simulink model "pi_IL_H2DF_2024a"  (R2024a)
settings: Solver=FixedStepAuto  StartTime=0.0  StopTime=inf  FixedStep=0.001  RelTol=1e-3  EnableMultiTasking=on
values from neighbouring files (symbols this model uses):
  IL = struct()    [init_simulink_IL_H2DF.m]
undefined symbols (not defined in the file or in its folder): C2C_NMPC
libraries: deeplib x1, raspberrypiNetworklib x1
(part 1 of 2)
settings Model: VariantConfigurationObject=C2C  SimulationMode=external  ExtModeTrigDuration=2  Creator=maxim  LastModifiedBy=winkler_a
settings SolverCC: PositivePriorityOrder=on
settings DataIOCC: LimitDataPoints=on  MaxDataPoints=10000  SaveOutput=off
settings OptimizationCC: EnhancedBackFolding=on  PassReuseOutputArgsAs=Individual arguments  ZeroExternalMemoryAtStartup=off  ZeroInternalMemoryAtStartup=off  MaxStackSize=64  OptimizeBlockOrder=speed  DifferentSizesBufferReuse=on  OptimizationCustomize=off  EfficientTunableParamExpr=on
settings DebuggingCC: ParameterTunabilityLossMsg=error
settings HardwareCC: ProdBitPerPointer=32  ProdBitPerSizeT=32  ProdBitPerPtrDiffT=32  ProdLargestAtomicInteger=Long  ProdLargestAtomicFloat=Double  ProdWordSize=32  ProdLongLongMode=on  ProdHWDeviceType=ARM Compatible->ARM Cortex
settings RTWCC: Description=Embedded Coder  SystemTargetFile=ert.tlc  HardwareBoard=Raspberry Pi  TemplateMakefile=ert_default_tmf  RTWUseSimCustomCode=on  Toolchain=GNU GCC Embedded Linux  BuildConfiguration=Faster Runs  GPUComputeCapability=3.5
settings CodeAppCC: ForceParamTrailComments=on  IgnoreCustomStorageClasses=off  OperatorAnnotations=on  SimulinkDataObjDesc=on  SFDataObjDesc=on  InsertBlockDesc=on
settings ERTTargetCC: SupportContinuousTime=on  SupportNonInlinedSFcns=on  SupportVariableSizeSignals=on  ExtMode=on  ExtModeStaticAlloc=on  ExtModeMaxTrigDuration=1000  ExtModeMexArgs='192.168.140.200' 0 17725

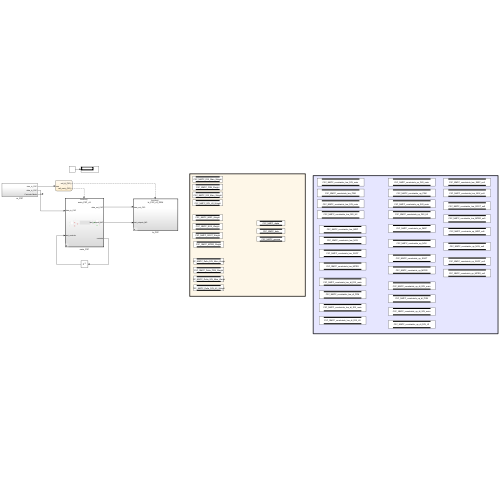
[thumbnail: Simulink's stored preview of the top-level diagram]
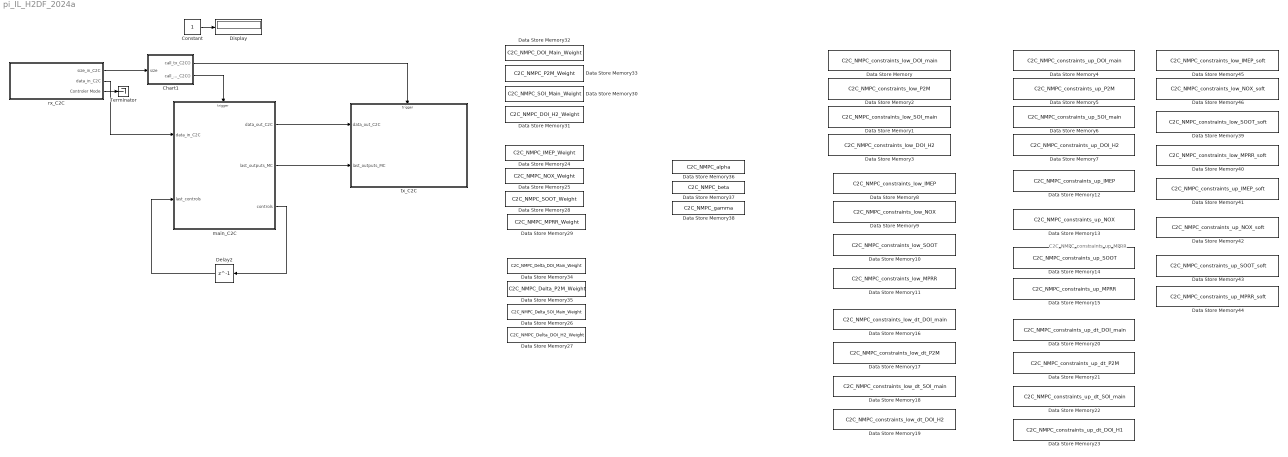
== system pi_IL_H2DF_2024a ==
  note: C2C_NMPC_constraints_up_MPRR
  Chart1 : Stateflow chart  TreatAsAtomicUnit=on
  Constant : Constant
  Data Store Memory : DataStoreMemory  DataStoreName=C2C_NMPC_constraints_low_DOI_main  WriteAfterWriteMsg=warning  ShowAdditionalParam=off
  Data Store Memory1 : DataStoreMemory  DataStoreName=C2C_NMPC_constraints_low_SOI_main  WriteAfterWriteMsg=warning  ShowAdditionalParam=off
  Data Store Memory10 : DataStoreMemory  DataStoreName=C2C_NMPC_constraints_low_SOOT  WriteAfterWriteMsg=warning  ShowAdditionalParam=off
  Data Store Memory11 : DataStoreMemory  DataStoreName=C2C_NMPC_constraints_low_MPRR  WriteAfterWriteMsg=warning  ShowAdditionalParam=off
  Data Store Memory12 : DataStoreMemory  DataStoreName=C2C_NMPC_constraints_up_IMEP  WriteAfterWriteMsg=warning  ShowAdditionalParam=off
  Data Store Memory13 : DataStoreMemory  DataStoreName=C2C_NMPC_constraints_up_NOX  WriteAfterWriteMsg=warning  ShowAdditionalParam=off
  Data Store Memory14 : DataStoreMemory  DataStoreName=C2C_NMPC_constraints_up_SOOT  WriteAfterWriteMsg=warning  ShowAdditionalParam=off
  Data Store Memory15 : DataStoreMemory  DataStoreName=C2C_NMPC_constraints_up_MPRR  WriteAfterWriteMsg=warning  ShowAdditionalParam=off
  Data Store Memory16 : DataStoreMemory  DataStoreName=C2C_NMPC_constraints_low_dt_DOI_main  WriteAfterWriteMsg=warning  ShowAdditionalParam=off
  Data Store Memory17 : DataStoreMemory  DataStoreName=C2C_NMPC_constraints_low_dt_P2M  WriteAfterWriteMsg=warning  ShowAdditionalParam=off
  Data Store Memory18 : DataStoreMemory  DataStoreName=C2C_NMPC_constraints_low_dt_SOI_main  WriteAfterWriteMsg=warning  ShowAdditionalParam=off
  Data Store Memory19 : DataStoreMemory  DataStoreName=C2C_NMPC_constraints_low_dt_DOI_H2  WriteAfterWriteMsg=warning  ShowAdditionalParam=off
  Data Store Memory2 : DataStoreMemory  DataStoreName=C2C_NMPC_constraints_low_P2M  WriteAfterWriteMsg=warning  ShowAdditionalParam=off
  Data Store Memory20 : DataStoreMemory  DataStoreName=C2C_NMPC_constraints_up_dt_DOI_main  WriteAfterWriteMsg=warning  ShowAdditionalParam=off
  Data Store Memory21 : DataStoreMemory  DataStoreName=C2C_NMPC_constraints_up_dt_P2M  WriteAfterWriteMsg=warning  ShowAdditionalParam=off
  Data Store Memory22 : DataStoreMemory  DataStoreName=C2C_NMPC_constraints_up_dt_SOI_main  WriteAfterWriteMsg=warning  ShowAdditionalParam=off
  Data Store Memory23 : DataStoreMemory  DataStoreName=C2C_NMPC_constraints_up_dt_DOI_H1  WriteAfterWriteMsg=warning  ShowAdditionalParam=off
  Data Store Memory24 : DataStoreMemory  DataStoreName=C2C_NMPC_IMEP_Weight  WriteAfterWriteMsg=warning  ShowAdditionalParam=off
  Data Store Memory25 : DataStoreMemory  DataStoreName=C2C_NMPC_NOX_Weight  WriteAfterWriteMsg=warning  ShowAdditionalParam=off
  Data Store Memory26 : DataStoreMemory  DataStoreName=C2C_NMPC_Delta_SOI_Main_Weight  WriteAfterWriteMsg=warning  ShowAdditionalParam=off
  Data Store Memory27 : DataStoreMemory  DataStoreName=C2C_NMPC_Delta_DOI_H2_Weight  WriteAfterWriteMsg=warning  ShowAdditionalParam=off
  Data Store Memory28 : DataStoreMemory  DataStoreName=C2C_NMPC_SOOT_Weight  WriteAfterWriteMsg=warning  ShowAdditionalParam=off
  Data Store Memory29 : DataStoreMemory  DataStoreName=C2C_NMPC_MPRR_Weight  WriteAfterWriteMsg=warning  ShowAdditionalParam=off
  Data Store Memory3 : DataStoreMemory  DataStoreName=C2C_NMPC_constraints_low_DOI_H2  WriteAfterWriteMsg=warning  ShowAdditionalParam=off
  Data Store Memory30 : DataStoreMemory  DataStoreName=C2C_NMPC_SOI_Main_Weight  WriteAfterWriteMsg=warning  ShowAdditionalParam=off
  Data Store Memory31 : DataStoreMemory  DataStoreName=C2C_NMPC_DOI_H2_Weight  WriteAfterWriteMsg=warning  ShowAdditionalParam=off
  Data Store Memory32 : DataStoreMemory  DataStoreName=C2C_NMPC_DOI_Main_Weight  WriteAfterWriteMsg=warning  ShowAdditionalParam=off
  Data Store Memory33 : DataStoreMemory  DataStoreName=C2C_NMPC_P2M_Weight  WriteAfterWriteMsg=warning  ShowAdditionalParam=off
  Data Store Memory34 : DataStoreMemory  DataStoreName=C2C_NMPC_Delta_DOI_Main_Weight  WriteAfterWriteMsg=warning  ShowAdditionalParam=off
  Data Store Memory35 : DataStoreMemory  DataStoreName=C2C_NMPC_Delta_P2M_Weight  WriteAfterWriteMsg=warning  ShowAdditionalParam=off
  Data Store Memory36 : DataStoreMemory  DataStoreName=C2C_NMPC_alpha  WriteAfterWriteMsg=warning  ShowAdditionalParam=off
  Data Store Memory37 : DataStoreMemory  DataStoreName=C2C_NMPC_beta  WriteAfterWriteMsg=warning  ShowAdditionalParam=off
  Data Store Memory38 : DataStoreMemory  DataStoreName=C2C_NMPC_gamma  WriteAfterWriteMsg=warning  ShowAdditionalParam=off
  Data Store Memory39 : DataStoreMemory  DataStoreName=C2C_NMPC_constraints_low_SOOT_soft  WriteAfterWriteMsg=warning  ShowAdditionalParam=off
  Data Store Memory4 : DataStoreMemory  DataStoreName=C2C_NMPC_constraints_up_DOI_main  WriteAfterWriteMsg=warning  ShowAdditionalParam=off
  Data Store Memory40 : DataStoreMemory  DataStoreName=C2C_NMPC_constraints_low_MPRR_soft  WriteAfterWriteMsg=warning  ShowAdditionalParam=off
  Data Store Memory41 : DataStoreMemory  DataStoreName=C2C_NMPC_constraints_up_IMEP_soft  WriteAfterWriteMsg=warning  ShowAdditionalParam=off
  Data Store Memory42 : DataStoreMemory  DataStoreName=C2C_NMPC_constraints_up_NOX_soft  WriteAfterWriteMsg=warning  ShowAdditionalParam=off
  Data Store Memory43 : DataStoreMemory  DataStoreName=C2C_NMPC_constraints_up_SOOT_soft  WriteAfterWriteMsg=warning  ShowAdditionalParam=off
  Data Store Memory44 : DataStoreMemory  DataStoreName=C2C_NMPC_constraints_up_MPRR_soft  WriteAfterWriteMsg=warning  ShowAdditionalParam=off
  Data Store Memory45 : DataStoreMemory  DataStoreName=C2C_NMPC_constraints_low_IMEP_soft  WriteAfterWriteMsg=warning  ShowAdditionalParam=off
  Data Store Memory46 : DataStoreMemory  DataStoreName=C2C_NMPC_constraints_low_NOX_soft  WriteAfterWriteMsg=warning  ShowAdditionalParam=off
  Data Store Memory5 : DataStoreMemory  DataStoreName=C2C_NMPC_constraints_up_P2M  WriteAfterWriteMsg=warning  ShowAdditionalParam=off
  Data Store Memory6 : DataStoreMemory  DataStoreName=C2C_NMPC_constraints_up_SOI_main  WriteAfterWriteMsg=warning  ShowAdditionalParam=off
  Data Store Memory7 : DataStoreMemory  DataStoreName=C2C_NMPC_constraints_up_DOI_H2  WriteAfterWriteMsg=warning  ShowAdditionalParam=off
  Data Store Memory8 : DataStoreMemory  DataStoreName=C2C_NMPC_constraints_low_IMEP  WriteAfterWriteMsg=warning  ShowAdditionalParam=off
  Data Store Memory9 : DataStoreMemory  DataStoreName=C2C_NMPC_constraints_low_NOX  WriteAfterWriteMsg=warning  ShowAdditionalParam=off
  Delay2 : Delay  DelayLength=1  InitialCondition=C2C_NMPC.x0([(C2C_NMPC.Dims.n_LSTM_states + 1):(C2C_NMPC.Dims.n_LSTM_states + C2C_NMPC.Dims.n_controls)])
  Display : Display
  Terminator : Terminator
  main_C2C : Subsystem  Variant=on  VariantControlMode=label  VariantControl=main_C2C_n3  LabelModeActiveChoice=main_C2C_n3
  rx_C2C : Subsystem
  tx_C2C : Subsystem  Variant=on  VariantControlMode=label  VariantControl=Choice  LabelModeActiveChoice=tx_C2C_n3_GRU
  wires:
  rx_C2C/1(size_in_C2C) -> Chart1/1(size)
  Chart1/1(call_tx_C2C()) -> tx_C2C/Trigger
  rx_C2C/2(data_in_C2C) -> main_C2C/1(data_in_C2C)
  Delay2/1 -> main_C2C/2(last_controls)
  Chart1/2(call_main_C2C()) -> main_C2C/Trigger
  main_C2C/1(data_out_C2C) -> tx_C2C/1(data_out_C2C)
  main_C2C/3(controls) -> Delay2/1
  main_C2C/2(last_outputs_MC) -> tx_C2C/2(last_outputs_MC)
  Constant/1 -> Display/1
  rx_C2C/3(Controler Mode) -> Terminator/1

== system pi_IL_H2DF_2024a/main_C2C ==
  data_in_C2C : Inport
  last_controls : Inport  Port=2
  function : TriggerPort  TriggerType=function-call  VariantControl=(inherit)
  main_C2C_n3 : Subsystem  VariantControl=main_C2C_n3
  data_out_C2C : Outport
  last_outputs_MC : Outport  Port=2
  controls : Outport  Port=3

== system pi_IL_H2DF_2024a/rx_C2C ==
  Data Type Conversion : DataTypeConversion  OutDataTypeStr=double  SaturateOnIntegerOverflow=off  RndMeth=Floor
  Receive : Subsystem
  UDP Receive1 : raspberrypiNetworklib/UDP Receive  localURL='0.0.0.0'  localPort=42785  remoteURL='0.0.0.0'  remotePort=-1  recvBufferSize=8192  signalDatatype=uint32  dims=56  isVarSize=off  showBlockingTime=off  blockingTime=0  sampletime=0.001  blockPlatform=Raspberry Pi
  size_in_C2C : Outport
  data_in_C2C : Outport  Port=2
  Controler Mode : Outport  Port=3
  wires:
  UDP Receive1/2 -> size_in_C2C/1
  UDP Receive1/1 -> Data Type Conversion/1
  Receive/1(udp_outputs) -> data_in_C2C/1
  Data Type Conversion/1 -> Receive/1(udp_data_in)
  Receive/2(controller_mode) -> Controler Mode/1

== system pi_IL_H2DF_2024a/tx_C2C ==
  data_out_C2C : Inport
  last_outputs_MC : Inport  Port=2
  function : TriggerPort  TriggerType=function-call  VariantControl=(inherit)
  tx_C2C_n3_GRU : Subsystem  VariantControl=tx_C2C_n3_GRU

== system pi_IL_H2DF_2024a/main_C2C/main_C2C_n3 ==
  data_in_C2C : Inport
  last_controls : Inport  Port=2
  function : TriggerPort  TriggerType=function-call  VariantControl=(inherit)
  Constant : Constant  Value=zeros(16,1)
  IC : InitialCondition  Value=C2C_NMPC.x0([(C2C_NMPC.Dims.n_LSTM_states + 1):(C2C_NMPC.Dims.n_LSTM_states + C2C_NMPC.Dims.n_controls)])
  IL_Controller : Subsystem  VariantControl=C2C_NMPC_n3
  Selector : Selector  InputPortWidth=C2C_NMPC.Dims.n_cost*3  IndexOptions=Index vector (dialog)  Indices=1:C2C_NMPC.Dims.n_cost  OutputSizes=1
  post_processing : Subsystem
  pre_processing1 : Subsystem
  data_out_C2C : Outport
  last_outputs_MC : Outport  Port=2
  controls : Outport  Port=3
  wires:
  post_processing/1(data_C2C_out) -> data_out_C2C/1
  pre_processing1/1(reference_C2C) -> IL_Controller/1(reference_C2C), Selector/1
  pre_processing1/2(counter_C2C) -> [counter_C2C]
  [counter_C2C] -> post_processing/5(counter)
  last_controls/1 -> [last_controls]
  IL_Controller/1(status_C2C) -> post_processing/3(controller_status)
  [last_outputs_MC] -> post_processing/4(last_outputs_MC)
  [last_outputs_MC] -> last_outputs_MC/1
  pre_processing1/3(last_outputs_MC) -> IL_Controller/2(last_outputs), [last_outputs_MC]
  data_in_C2C/1 -> pre_processing1/1(data_in_C2C)
  Selector/1 -> post_processing/1(reference)
  IL_Controller/2(controls) -> IC/1
  IC/1 -> post_processing/2(controls), controls/1
  Constant/1 -> post_processing/6(LSTM_States)

== system pi_IL_H2DF_2024a/rx_C2C/Receive ==
  note: block for horizon of 3 from engine
  udp_data_in : Inport
  conversion_n3 : Subsystem
  udp_outputs : Outport
  controller_mode : Outport  Port=2
  wires:
  udp_data_in/1 -> conversion_n3/1(udp_data_in)
  conversion_n3/1(udp_outputs) -> udp_outputs/1
  conversion_n3/2(controller_mode) -> controller_mode/1

== system pi_IL_H2DF_2024a/tx_C2C/tx_C2C_n3_GRU ==
  note: [1:4,13,99:134,14,15,16,17,71:74]
  data_out_C2C : Inport
  last_outputs_MC : Inport  Port=2
  function : TriggerPort  TriggerType=function-call  VariantControl=(inherit)
  Data Type Conversion : DataTypeConversion  OutDataTypeStr=uint32  SaturateOnIntegerOverflow=off  RndMeth=Floor
  Selector : Selector  IndexOptions=Index vector (dialog)  Indices=[1:4,13,115:142,14,15,16,17,95:98]  OutputSizes=1
  Subsystem : Subsystem
  UDP Send1 : S-Function  AncestorBlock=raspberrypiNetworklib/UDP Send  InitFcn=|  FunctionName=sdspToNetwork  Parameters=localURL, localPortSource, localPort, remoteURL, remotePort, 8192, separateLengthPort, []  SFunctionDeploymentMode=off  EnableBusSupport=off  mask(UDP Send){remoteURL='192.168.140.159', remotePort=42784, localURL='0.0.0.0', localPortSource=Specify via dialog, localPort=42784, sampletime=-1, blockPlatform=Raspberry Pi, separateLengthPort=0}
      | realtime.internal.validateLinuxBlock(get_param(gcbh, 'blockPlatform'), gcbh);
      | realtime.internal.registerLinuxBlock(gcb);
      mask prompts: remoteURL "Remote IP address ('255.255.255.255' for broadcast):"; remotePort "Remote IP port:"; localURL "Local IP address:"; localPortSource "Local IP port source:"; localPort "Local IP port:"; blockPlatform "Block Platform"; separateLengthPort "Use a separate length port"
      mask help: Sends UDP packets to another UDP host on an Internet network. Set Remote IP address parameter to the IP address of the receiving UDP host. Set the Remote IP port parameter to the port number used by the receiving UDP host.
      settings: LibrarySourceBlock=raspberrypiNetworklib/UDP Send
      mask Help: eval('realtime.helpView(get_param(gcb, ''blockPlatform''), [realtime.internal.getHelpLinkPrefix(gcb) ''libudpsend''])');
      mask TypeOptions localPortSource: Automatically determine | Specify via dialog
      mask Callback localPortSource:
      | mask_vis = get_param(gcbh, 'MaskVisibilities');
      | if strcmp(get_param(gcbh,'localPortSource'),'Specify via dialog')
      |     mask_vis{5} = 'on';
      | else
      |     mask_vis{5} = 'off';
      | end
      | set_param(gcbh, 'MaskVisibilities', mask_vis);
      | clear('mask_vis');
      mask Display:
      | %fprintf('UDP Send');
      | color('blue');
      | [data, map]=imread('ethernet2_bw.gif');pic=ind2rgb(data,map);image(pic,[0.32 0.25 0.40 0.45]);
      | platform = realtime.internal.getBlockDisplayText(gcb);
      | text(0.99, 0.9, platform, 'horizontalalignment', 'right');
  wires:
  data_out_C2C/1 -> Selector/1
  Data Type Conversion/1 -> UDP Send1/1
  Subsystem/1(Out1) -> Data Type Conversion/1
  Selector/1 -> Subsystem/1(In1)

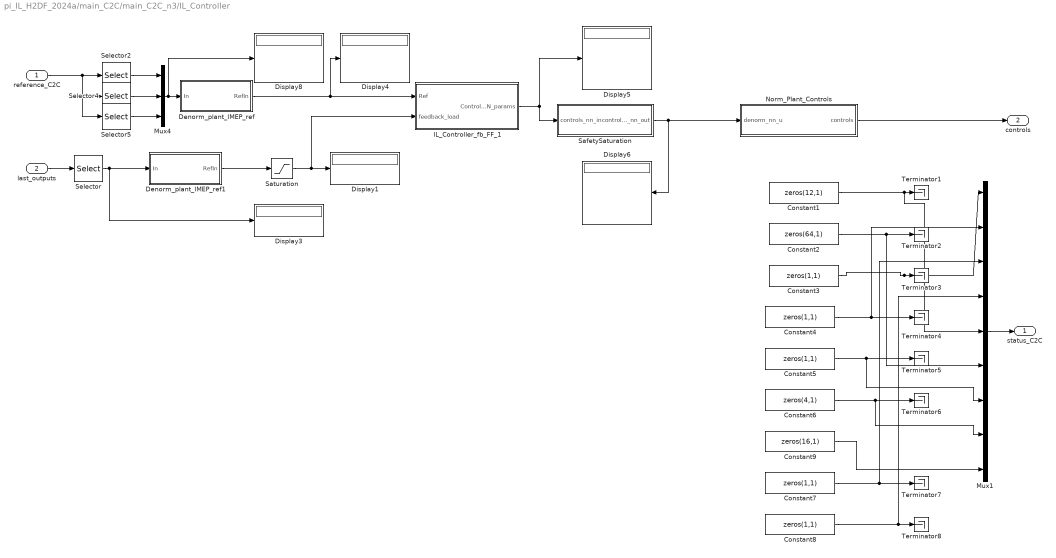
== system pi_IL_H2DF_2024a/main_C2C/main_C2C_n3/IL_Controller ==
  reference_C2C : Inport
  last_outputs : Inport  Port=2
  Constant1 : Constant  Value=zeros(12,1)
  Constant2 : Constant  Value=zeros(64,1)
  Constant{3..5,7..8} (5 alike) : Constant  Value=zeros(1,1)
  Constant6 : Constant  Value=zeros(4,1)
  Constant9 : Constant  Value=zeros(16,1)
  Denorm_plant_IMEP_ref : Subsystem
  Denorm_plant_IMEP_ref1 : Subsystem
  Display{1,3..6,8} (6 alike) : Display
  IL_Controller_fb_FF_1 : Subsystem  VariantControl=fb_LSTM_321_syn
  Mux1 : Mux  Inputs=9
  Mux4 : Mux  Inputs=3
  Norm_Plant_Controls : Subsystem
  SafetySaturation : Subsystem
  Saturation : Saturate  UpperLimit=8.5e5  LowerLimit=3e5
  Selector : Selector  InputPortWidth=4  IndexOptions=Index vector (dialog)  Indices=[1]  OutputSizes=1
  Selector2 : Selector  IndexOptions=Index vector (dialog)  Indices=5  OutputSizes=1
  Selector4 : Selector  IndexOptions=Index vector (dialog)  Indices=[ (C2C_NMPC.Dims.n_cost + 5) : (C2C_NMPC.Dims.n_cost + 5) ]  OutputSizes=1
  Selector5 : Selector  IndexOptions=Index vector (dialog)  Indices=[ (C2C_NMPC.Dims.n_cost * 2 + 5) : (C2C_NMPC.Dims.n_cost * 2 + 5 ) ]  OutputSizes=1
  Terminator{1..8} (8 alike) : Terminator
  status_C2C : Outport
  controls : Outport  Port=2
  wires:
  Constant4/1 -> Mux1/2, Terminator4/1
  Mux1/1 -> status_C2C/1
  SafetySaturation/1(controls_nn_out) -> Norm_Plant_Controls/1(denorm_nn_u), Display6/1
  Constant8/1 -> Terminator8/1, Mux1/4
  Constant7/1 -> Terminator7/1, Mux1/3
  Constant6/1 -> Terminator6/1, Mux1/8
  Constant5/1 -> Terminator5/1, Mux1/7
  Constant9/1 -> Mux1/9
  Constant3/1 -> Mux1/1, Terminator3/1
  Constant2/1 -> Terminator2/1, Mux1/6
  Constant1/1 -> Terminator1/1, Mux1/5
  IL_Controller_fb_FF_1/1(Control_norm_NN_params) -> Display5/1, SafetySaturation/1(controls_nn_in)
  Selector4/1 -> Mux4/2
  Selector2/1 -> Mux4/1
  Selector5/1 -> Mux4/3
  Mux4/1 -> Denorm_plant_IMEP_ref/1(In), Display8/1
  Saturation/1 -> IL_Controller_fb_FF_1/2(feedback_load), Display1/1
  reference_C2C/1 -> Selector5/1, Selector4/1, Selector2/1
  last_outputs/1 -> Selector/1
  Selector/1 -> Denorm_plant_IMEP_ref1/1(In), Display3/1
  Denorm_plant_IMEP_ref/1(RefIn) -> IL_Controller_fb_FF_1/1(Ref), Display4/1
  Norm_Plant_Controls/1(controls) -> controls/1
  Denorm_plant_IMEP_ref1/1(RefIn) -> Saturation/1

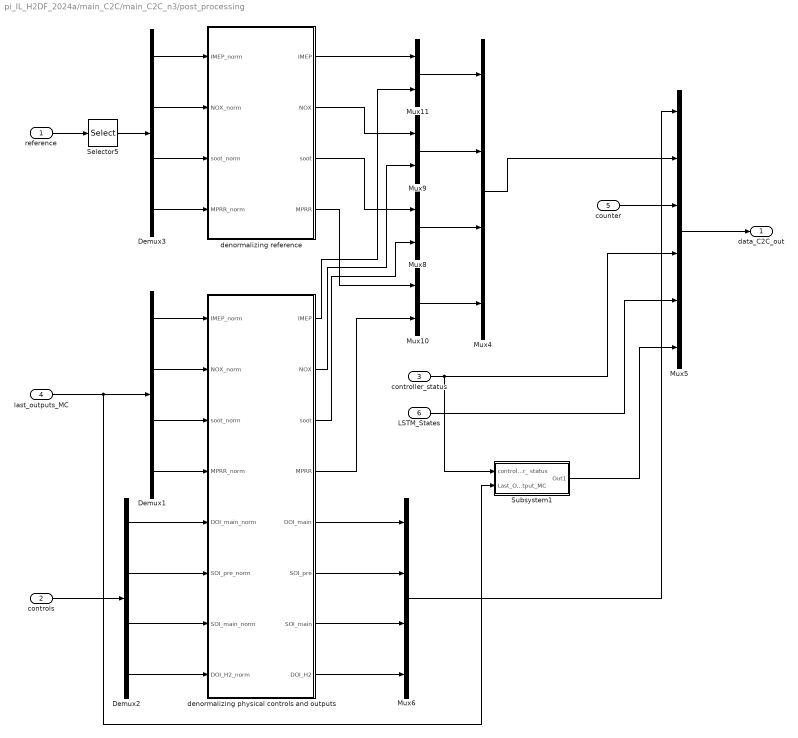
== system pi_IL_H2DF_2024a/main_C2C/main_C2C_n3/post_processing ==
  reference : Inport
  controls : Inport  Port=2
  controller_status : Inport  Port=3
  last_outputs_MC : Inport  Port=4
  counter : Inport  Port=5
  LSTM_States : Inport  Port=6
  " denormalizing reference" : Subsystem
  Demux1 : Demux
  Demux2 : Demux
  Demux3 : Demux
  Mux{8..11} (4 alike) : Mux  Inputs=2
  Mux4 : Mux
  Mux5 : Mux  Inputs=6
  Mux6 : Mux
  Selector5 : Selector  IndexOptions=Index vector (dialog)  Indices=[(C2C_NMPC.Dims.n_controls + 1 ):(C2C_NMPC.Dims.n_cost - C2C_NMPC.Dims.n_controls)]  OutputSizes=1
  Subsystem1 : Subsystem
  denormalizing physical controls and outputs : Subsystem
  data_C2C_out : Outport
  wires:
  Demux3/1 -> " denormalizing reference"/1(IMEP_norm)
  Demux3/2 -> " denormalizing reference"/2(NOX_norm)
  Demux3/4 -> " denormalizing reference"/4(MPRR_norm)
  Demux3/3 -> " denormalizing reference"/3(soot_norm)
  reference/1 -> Selector5/1
  Selector5/1 -> Demux3/1
  controls/1 -> Demux2/1
  Demux1/1 -> denormalizing physical controls and outputs/1(IMEP_norm)
  Demux1/2 -> denormalizing physical controls and outputs/2(NOX_norm)
  Demux1/3 -> denormalizing physical controls and outputs/3(soot_norm)
  Demux1/4 -> denormalizing physical controls and outputs/4(MPRR_norm)
  Demux2/1 -> denormalizing physical controls and outputs/5(DOI_main_norm)
  Demux2/2 -> denormalizing physical controls and outputs/6(SOI_pre_norm)
  Demux2/3 -> denormalizing physical controls and outputs/7(SOI_main_norm)
  denormalizing physical controls and outputs/5(DOI_main) -> Mux6/1
  denormalizing physical controls and outputs/6(SOI_pre) -> Mux6/2
  denormalizing physical controls and outputs/7(SOI_main) -> Mux6/3
  " denormalizing reference"/1(IMEP) -> Mux11/1
  " denormalizing reference"/2(NOX) -> Mux9/1
  " denormalizing reference"/3(soot) -> Mux8/1
  " denormalizing reference"/4(MPRR) -> Mux10/1
  controller_status/1 -> Mux5/4, Subsystem1/1(controller_ status)
  Mux5/1 -> data_C2C_out/1
  Mux11/1 -> Mux4/1
  Mux8/1 -> Mux4/3
  Mux10/1 -> Mux4/4
  denormalizing physical controls and outputs/1(IMEP) -> Mux11/2
  denormalizing physical controls and outputs/2(NOX) -> Mux9/2
  denormalizing physical controls and outputs/3(soot) -> Mux8/2
  denormalizing physical controls and outputs/4(MPRR) -> Mux10/2
  Mux4/1 -> Mux5/2
  counter/1 -> Mux5/3
  Mux6/1 -> Mux5/1
  Demux2/4 -> denormalizing physical controls and outputs/8(DOI_H2_norm)
  denormalizing physical controls and outputs/8(DOI_H2) -> Mux6/4
  Mux9/1 -> Mux4/2
  LSTM_States/1 -> Mux5/5
  last_outputs_MC/1 -> Subsystem1/2(Last_Output_MC), Demux1/1
  Subsystem1/1(Out1) -> Mux5/6

== system pi_IL_H2DF_2024a/main_C2C/main_C2C_n3/pre_processing1 ==
  data_in_C2C : Inport
  Selector : Selector  IndexOptions=Index vector (dialog)  Indices=[6]  OutputSizes=1
  normalize_last_outputs_MC : Subsystem
  normalize_reference_C2C : Subsystem
  reference_C2C : Outport  VectorParamsAs1DForOutWhenUnconnected=off
  counter_C2C : Outport  Port=2  VectorParamsAs1DForOutWhenUnconnected=off
  last_outputs_MC : Outport  Port=3  VectorParamsAs1DForOutWhenUnconnected=off
  wires:
  normalize_reference_C2C/1(reference_C2C) -> reference_C2C/1
  data_in_C2C/1 -> Selector/1, normalize_last_outputs_MC/1(data_in), normalize_reference_C2C/1(data_in)
  normalize_last_outputs_MC/1(last_outputs_MC) -> last_outputs_MC/1
  Selector/1 -> counter_C2C/1

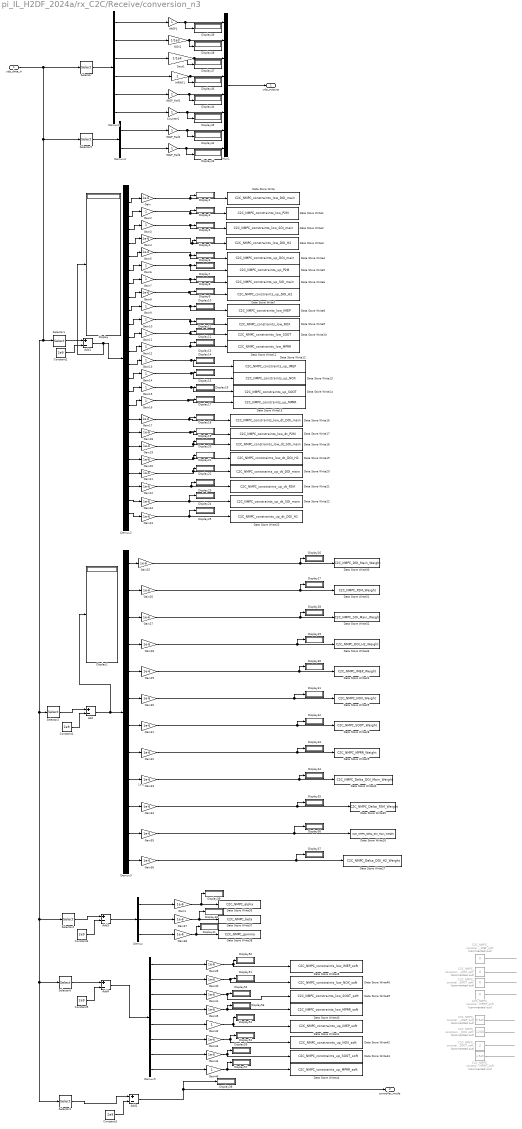
== system pi_IL_H2DF_2024a/rx_C2C/Receive/conversion_n3 ==
  note: 1e-6
  udp_data_in : Inport
  Add{,1..4} (5 alike) : Sum  Inputs=+-
  C2C_NMPC_constraints_low_IMEP_soft : Constant  Commented=on  Value=0
  C2C_NMPC_constraints_low_MPRR_soft : Constant  Commented=on  Value=0
  C2C_NMPC_constraints_low_NOX_soft : Constant  Commented=on  Value=0
  C2C_NMPC_constraints_low_SOOT_soft : Constant  Commented=on  Value=0
  C2C_NMPC_constraints_up_IMEP_soft : Constant  Commented=on  Value=9.5e5
  C2C_NMPC_constraints_up_MPRR_soft : Constant  Commented=on  Value=4.5e5
  C2C_NMPC_constraints_up_NOX_soft : Constant  Commented=on  Value=1200
  C2C_NMPC_constraints_up_SOOT_soft : Constant  Commented=on  Value=2
  Constant{1..5} (5 alike) : Constant  Value=2e9
  Counter1 : Gain
  Data Store Write : DataStoreWrite  DataStoreName=C2C_NMPC_constraints_low_DOI_main  IndexOptions=Index vector (dialog)  Indices=1  OutputSizes=1
  Data Store Write1 : DataStoreWrite  DataStoreName=C2C_NMPC_constraints_low_P2M  IndexOptions=Index vector (dialog)  Indices=1  OutputSizes=1
  Data Store Write10 : DataStoreWrite  DataStoreName=C2C_NMPC_constraints_low_SOOT  IndexOptions=Index vector (dialog)  Indices=1  OutputSizes=1
  Data Store Write11 : DataStoreWrite  DataStoreName=C2C_NMPC_constraints_low_MPRR  IndexOptions=Index vector (dialog)  Indices=1  OutputSizes=1
  Data Store Write12 : DataStoreWrite  DataStoreName=C2C_NMPC_constraints_up_IMEP  IndexOptions=Index vector (dialog)  Indices=1  OutputSizes=1
  Data Store Write13 : DataStoreWrite  DataStoreName=C2C_NMPC_constraints_up_NOX  IndexOptions=Index vector (dialog)  Indices=1  OutputSizes=1
  Data Store Write14 : DataStoreWrite  DataStoreName=C2C_NMPC_constraints_up_SOOT  IndexOptions=Index vector (dialog)  Indices=1  OutputSizes=1
  Data Store Write15 : DataStoreWrite  DataStoreName=C2C_NMPC_constraints_up_MPRR  IndexOptions=Index vector (dialog)  Indices=1  OutputSizes=1
  Data Store Write16 : DataStoreWrite  DataStoreName=C2C_NMPC_constraints_low_dt_DOI_main  IndexOptions=Index vector (dialog)  Indices=1  OutputSizes=1
  Data Store Write17 : DataStoreWrite  DataStoreName=C2C_NMPC_constraints_low_dt_P2M  IndexOptions=Index vector (dialog)  Indices=1  OutputSizes=1
  Data Store Write18 : DataStoreWrite  DataStoreName=C2C_NMPC_constraints_low_dt_SOI_main  IndexOptions=Index vector (dialog)  Indices=1  OutputSizes=1
  Data Store Write19 : DataStoreWrite  DataStoreName=C2C_NMPC_constraints_low_dt_DOI_H2  IndexOptions=Index vector (dialog)  Indices=1  OutputSizes=1
  Data Store Write2 : DataStoreWrite  DataStoreName=C2C_NMPC_constraints_low_SOI_main  IndexOptions=Index vector (dialog)  Indices=1  OutputSizes=1
  Data Store Write20 : DataStoreWrite  DataStoreName=C2C_NMPC_constraints_up_dt_DOI_main  IndexOptions=Index vector (dialog)  Indices=1  OutputSizes=1
  Data Store Write21 : DataStoreWrite  DataStoreName=C2C_NMPC_constraints_up_dt_P2M  IndexOptions=Index vector (dialog)  Indices=1  OutputSizes=1
  Data Store Write22 : DataStoreWrite  DataStoreName=C2C_NMPC_constraints_up_dt_SOI_main  IndexOptions=Index vector (dialog)  Indices=1  OutputSizes=1
  Data Store Write23 : DataStoreWrite  DataStoreName=C2C_NMPC_constraints_up_dt_DOI_H1  IndexOptions=Index vector (dialog)  Indices=1  OutputSizes=1
  Data Store Write24 : DataStoreWrite  DataStoreName=C2C_NMPC_IMEP_Weight  IndexOptions=Index vector (dialog)  Indices=1  OutputSizes=1
  Data Store Write25 : DataStoreWrite  DataStoreName=C2C_NMPC_NOX_Weight  IndexOptions=Index vector (dialog)  Indices=1  OutputSizes=1
  Data Store Write26 : DataStoreWrite  DataStoreName=C2C_NMPC_Delta_SOI_Main_Weight  IndexOptions=Index vector (dialog)  Indices=1  OutputSizes=1
  Data Store Write27 : DataStoreWrite  DataStoreName=C2C_NMPC_Delta_DOI_H2_Weight  IndexOptions=Index vector (dialog)  Indices=1  OutputSizes=1
  Data Store Write28 : DataStoreWrite  DataStoreName=C2C_NMPC_SOOT_Weight  IndexOptions=Index vector (dialog)  Indices=1  OutputSizes=1
  Data Store Write29 : DataStoreWrite  DataStoreName=C2C_NMPC_MPRR_Weight  IndexOptions=Index vector (dialog)  Indices=1  OutputSizes=1
  Data Store Write3 : DataStoreWrite  DataStoreName=C2C_NMPC_constraints_low_DOI_H2  IndexOptions=Index vector (dialog)  Indices=1  OutputSizes=1
  Data Store Write30 : DataStoreWrite  DataStoreName=C2C_NMPC_DOI_Main_Weight  IndexOptions=Index vector (dialog)  Indices=1  OutputSizes=1
  Data Store Write31 : DataStoreWrite  DataStoreName=C2C_NMPC_P2M_Weight  IndexOptions=Index vector (dialog)  Indices=1  OutputSizes=1
  Data Store Write32 : DataStoreWrite  DataStoreName=C2C_NMPC_SOI_Main_Weight  IndexOptions=Index vector (dialog)  Indices=1  OutputSizes=1
  Data Store Write33 : DataStoreWrite  DataStoreName=C2C_NMPC_DOI_H2_Weight  IndexOptions=Index vector (dialog)  Indices=1  OutputSizes=1
  Data Store Write34 : DataStoreWrite  DataStoreName=C2C_NMPC_Delta_DOI_Main_Weight  IndexOptions=Index vector (dialog)  Indices=1  OutputSizes=1
  Data Store Write35 : DataStoreWrite  DataStoreName=C2C_NMPC_Delta_P2M_Weight  IndexOptions=Index vector (dialog)  Indices=1  OutputSizes=1
  Data Store Write36 : DataStoreWrite  DataStoreName=C2C_NMPC_alpha  IndexOptions=Index vector (dialog)  Indices=1  OutputSizes=1
  Data Store Write37 : DataStoreWrite  DataStoreName=C2C_NMPC_beta  IndexOptions=Index vector (dialog)  Indices=1  OutputSizes=1
  Data Store Write38 : DataStoreWrite  DataStoreName=C2C_NMPC_gamma  IndexOptions=Index vector (dialog)  Indices=1  OutputSizes=1
  Data Store Write39 : DataStoreWrite  DataStoreName=C2C_NMPC_constraints_low_SOOT_soft  IndexOptions=Index vector (dialog)  Indices=1  OutputSizes=1
  Data Store Write4 : DataStoreWrite  DataStoreName=C2C_NMPC_constraints_up_DOI_main  IndexOptions=Index vector (dialog)  Indices=1  OutputSizes=1
  Data Store Write40 : DataStoreWrite  DataStoreName=C2C_NMPC_constraints_low_MPRR_soft  IndexOptions=Index vector (dialog)  Indices=1  OutputSizes=1
  Data Store Write41 : DataStoreWrite  DataStoreName=C2C_NMPC_constraints_up_IMEP_soft  IndexOptions=Index vector (dialog)  Indices=1  OutputSizes=1
  Data Store Write42 : DataStoreWrite  DataStoreName=C2C_NMPC_constraints_up_NOX_soft  IndexOptions=Index vector (dialog)  Indices=1  OutputSizes=1
  Data Store Write43 : DataStoreWrite  DataStoreName=C2C_NMPC_constraints_up_SOOT_soft  IndexOptions=Index vector (dialog)  Indices=1  OutputSizes=1
  Data Store Write44 : DataStoreWrite  DataStoreName=C2C_NMPC_constraints_up_MPRR_soft  IndexOptions=Index vector (dialog)  Indices=1  OutputSizes=1
  Data Store Write45 : DataStoreWrite  DataStoreName=C2C_NMPC_constraints_low_IMEP_soft  IndexOptions=Index vector (dialog)  Indices=1  OutputSizes=1
  Data Store Write46 : DataStoreWrite  DataStoreName=C2C_NMPC_constraints_low_NOX_soft  IndexOptions=Index vector (dialog)  Indices=1  OutputSizes=1
  Data Store Write5 : DataStoreWrite  DataStoreName=C2C_NMPC_constraints_up_P2M  IndexOptions=Index vector (dialog)  Indices=1  OutputSizes=1
  Data Store Write6 : DataStoreWrite  DataStoreName=C2C_NMPC_constraints_up_SOI_main  IndexOptions=Index vector (dialog)  Indices=1  OutputSizes=1
  Data Store Write7 : DataStoreWrite  DataStoreName=C2C_NMPC_constraints_up_DOI_H2  IndexOptions=Index vector (dialog)  Indices=1  OutputSizes=1
  Data Store Write8 : DataStoreWrite  DataStoreName=C2C_NMPC_constraints_low_IMEP  IndexOptions=Index vector (dialog)  Indices=1  OutputSizes=1
  Data Store Write9 : DataStoreWrite  DataStoreName=C2C_NMPC_constraints_low_NOX  IndexOptions=Index vector (dialog)  Indices=1  OutputSizes=1
  Demux : Demux  Outputs=3
  Demux1 : Demux  Outputs=6
  Demux2 : Demux  Outputs=24
  Demux3 : Demux  Outputs=12
  Demux4 : Demux  Outputs=2
  Demux5 : Demux  Outputs=8
  Display{,1..57} (58 alike) : Display
  Gain{,1,4..5,8,17..41,43..45} (33 alike) : Gain  Gain=1e-6
  Gain{2..3,6..7,9..16,42,46} (14 alike) : Gain
  IMEP1 : Gain
  IMEP_Ref1 : Gain
  IMEP_Ref2 : Gain
  IMEP_Ref3 : Gain
  MPRR1 : Gain
  Mux1 : Mux  Inputs=8
  NOX1 : Gain  Gain=1/1e3
  Selector : Selector  IndexOptions=Index vector (dialog)  Indices=[1:6]  OutputSizes=1
  Selector1 : Selector  IndexOptions=Index vector (dialog)  Indices=[7:30]  OutputSizes=1
  Selector2 : Selector  IndexOptions=Index vector (dialog)  Indices=[31:42]  OutputSizes=1
  Selector3 : Selector  IndexOptions=Index vector (dialog)  Indices=[54]  OutputSizes=1
  Selector4 : Selector  IndexOptions=Index vector (dialog)  Indices=[43:45]  OutputSizes=1
  Selector5 : Selector  IndexOptions=Index vector (dialog)  Indices=[55:56]  OutputSizes=1
  Selector6 : Selector  IndexOptions=Index vector (dialog)  Indices=[46:53]  OutputSizes=1
  Soot1 : Gain  Gain=1/1e4
  udp_outputs : Outport
  controller_mode : Outport  Port=2
  wires:
  Demux2/16 -> Gain16/1
  Demux2/1 -> Gain/1
  Demux3/9 -> Gain33/1
  Demux2/9 -> Gain9/1
  Demux2/2 -> Gain2/1
  Demux3/11 -> Gain35/1
  Demux1/1 -> IMEP1/1
  Demux2/3 -> Gain3/1
  Demux2/23 -> Gain24/1
  Demux2/18 -> Gain18/1
  Demux3/2 -> Gain26/1
  Demux1/2 -> NOX1/1
  Demux2/12 -> Gain12/1
  Demux2/19 -> Gain19/1
  Demux2/21 -> Gain21/1
  Demux1/3 -> Soot1/1
  Demux3/3 -> Gain27/1
  Demux2/15 -> Gain15/1
  Demux2/7 -> Gain7/1
  Demux3/10 -> Gain34/1
  Demux2/10 -> Gain10/1
  Demux3/8 -> Gain32/1
  Demux2/4 -> Gain4/1
  Demux2/22 -> Gain22/1
  Demux2/13 -> Gain13/1
  Demux2/14 -> Gain14/1
  Demux2/20 -> Gain20/1
  Demux2/11 -> Gain11/1
  Demux2/5 -> Gain5/1
  Selector/1 -> Demux1/1
  Demux3/6 -> Gain30/1
  Demux2/6 -> Gain6/1
  Mux1/1 -> udp_outputs/1
  Demux2/17 -> Gain17/1
  Demux2/24 -> Gain23/1
  Demux2/8 -> Gain8/1
  Demux3/4 -> Gain28/1
  Demux1/4 -> MPRR1/1
  Demux3/7 -> Gain31/1
  Demux3/1 -> Gain25/1
  Demux1/6 -> Counter1/1
  Counter1/1 -> Display45/1, Mux1/6
  NOX1/1 -> Display48/1, Mux1/2
  Soot1/1 -> Display47/1, Mux1/3
  Demux3/12 -> Gain36/1
  Demux1/5 -> IMEP_Ref1/1
  IMEP1/1 -> Display49/1, Mux1/1
  Demux3/5 -> Gain29/1
  Add/1 -> Display1/1, Demux3/1
  Constant1/1 -> Add/2
  Gain/1 -> Display2/1, Data Store Write/1
  Gain2/1 -> Display3/1, Data Store Write1/1
  Gain3/1 -> Data Store Write2/1, Display5/1
  Gain4/1 -> Display4/1, Data Store Write3/1
  Gain5/1 -> Display6/1, Data Store Write4/1
  Gain6/1 -> Display7/1, Data Store Write5/1
  Gain7/1 -> Display8/1, Data Store Write6/1
  Gain8/1 -> Display9/1, Data Store Write7/1
  Gain9/1 -> Display10/1, Data Store Write8/1
  Gain10/1 -> Display11/1, Data Store Write9/1
  Gain11/1 -> Display12/1, Data Store Write10/1
  Gain12/1 -> Display13/1, Data Store Write11/1
  Gain13/1 -> Data Store Write12/1, Display14/1
  Gain14/1 -> Display15/1, Data Store Write13/1
  Gain15/1 -> Data Store Write14/1, Display16/1
  Gain16/1 -> Display17/1, Data Store Write15/1
  Gain17/1 -> Display18/1, Data Store Write16/1
  Gain18/1 -> Display19/1, Data Store Write17/1
  Gain19/1 -> Display20/1, Data Store Write18/1
  Gain20/1 -> Display21/1, Data Store Write19/1
  Gain21/1 -> Display22/1, Data Store Write20/1
  Gain22/1 -> Display23/1, Data Store Write21/1
  Gain23/1 -> Display25/1, Data Store Write23/1
  Gain24/1 -> Display24/1, Data Store Write22/1
  Gain25/1 -> Display26/1, Data Store Write30/1
  Gain26/1 -> Display27/1, Data Store Write31/1
  Gain27/1 -> Display28/1, Data Store Write32/1
  Gain28/1 -> Display29/1, Data Store Write33/1
  Gain29/1 -> Display30/1, Data Store Write24/1
  Gain30/1 -> Display31/1, Data Store Write25/1
  Gain31/1 -> Display32/1, Data Store Write28/1
  Gain32/1 -> Display33/1, Data Store Write29/1
  Gain33/1 -> Display34/1, Data Store Write34/1
  Gain34/1 -> Display35/1, Data Store Write35/1
  Gain35/1 -> Display36/1, Data Store Write26/1
  Gain36/1 -> Display37/1, Data Store Write27/1
  Selector2/1 -> Add/1
  Selector1/1 -> Add1/1
  Add1/1 -> Display/1, Demux2/1
  Constant2/1 -> Add1/2
  Constant3/1 -> Add2/2
  Selector3/1 -> Add2/1
  Add2/1 -> controller_mode/1, Display38/1
  Constant4/1 -> Add3/2
  Selector4/1 -> Add3/1
  Add3/1 -> Demux/1
  Demux/1 -> Gain1/1
  Demux/2 -> Gain37/1
  Demux/3 -> Gain38/1
  Gain37/1 -> Display40/1, Data Store Write37/1
  Gain1/1 -> Display39/1, Data Store Write36/1
  Gain38/1 -> Display41/1, Data Store Write38/1
  IMEP_Ref2/1 -> Display42/1, Mux1/7
  IMEP_Ref3/1 -> Display43/1, Mux1/8
  Selector5/1 -> Demux4/1
  Demux4/2 -> IMEP_Ref3/1
  Demux4/1 -> IMEP_Ref2/1
  IMEP_Ref1/1 -> Mux1/5, Display44/1
  C2C_NMPC_constraints_low_SOOT_soft/1 -> ?
  C2C_NMPC_constraints_up_SOOT_soft/1 -> ?
  C2C_NMPC_constraints_up_MPRR_soft/1 -> ?
  C2C_NMPC_constraints_low_NOX_soft/1 -> ?
  C2C_NMPC_constraints_low_MPRR_soft/1 -> ?
  C2C_NMPC_constraints_up_NOX_soft/1 -> ?
  C2C_NMPC_constraints_up_IMEP_soft/1 -> ?
  C2C_NMPC_constraints_low_IMEP_soft/1 -> ?
  Gain41/1 -> Data Store Write39/1, Display52/1
  Gain39/1 -> Data Store Write45/1, Display50/1
  Gain40/1 -> Display51/1, Data Store Write46/1
  Demux5/3 -> Gain41/1
  Demux5/2 -> Gain40/1
  Demux5/1 -> Gain39/1
  Add4/1 -> Demux5/1
  Selector6/1 -> Add4/1
  Constant5/1 -> Add4/2
  udp_data_in/1 -> Selector5/1, Selector3/1, Selector6/1, Selector4/1, Selector2/1, Selector1/1, Selector/1
  Gain43/1 -> Data Store Write42/1, Display54/1
  Gain42/1 -> Display53/1, Data Store Write41/1
  Gain44/1 -> Data Store Write43/1, Display55/1
  Gain45/1 -> Display56/1, Data Store Write40/1
  Gain46/1 -> Data Store Write44/1, Display57/1
  Demux5/4 -> Gain45/1
  Demux5/5 -> Gain42/1
  Demux5/6 -> Gain43/1
  Demux5/7 -> Gain44/1
  Demux5/8 -> Gain46/1
  MPRR1/1 -> Display46/1, Mux1/4

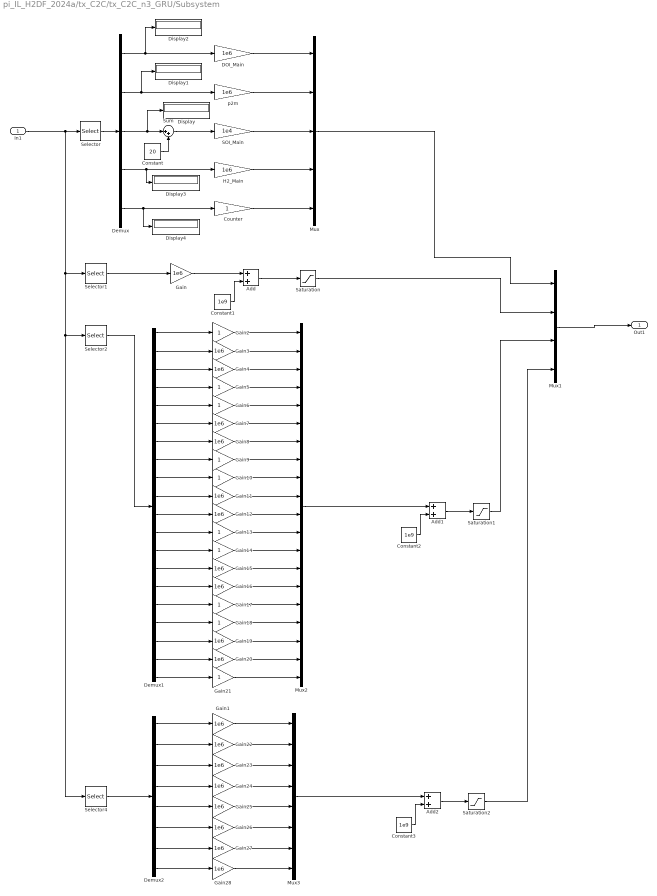
== system pi_IL_H2DF_2024a/tx_C2C/tx_C2C_n3_GRU/Subsystem ==
  In1 : Inport
  Add : Sum
  Add1 : Sum
  Add2 : Sum
  Constant : Constant  Value=20
  Constant1 : Constant  Value=1e9
  Constant2 : Constant  Value=1e9
  Constant3 : Constant  Value=1e9
  Counter : Gain
  DOI_Main : Gain  Gain=1e6
  Demux : Demux  Outputs=5
  Demux1 : Demux  Outputs=20
  Demux2 : Demux  Outputs=8
  Display{,1..4} (5 alike) : Display
  Gain{,1,3..4,7..8,11..12,15..16,19..20,22..28} (19 alike) : Gain  Gain=1e6
  Gain{2,5..6,9..10,13..14,17..18,21} (10 alike) : Gain
  H2_Main : Gain  Gain=1e6
  Mux : Mux  Inputs=5
  Mux1 : Mux
  Mux2 : Mux  Inputs=20
  Mux3 : Mux  Inputs=8
  SOI_Main : Gain  Gain=1e4
  Saturation : Saturate  UpperLimit=4e9  LowerLimit=0
  Saturation1 : Saturate  UpperLimit=4e9  LowerLimit=0
  Saturation2 : Saturate  UpperLimit=4e9  LowerLimit=0
  Selector : Selector  IndexOptions=Index vector (dialog)  Indices=[1:5]  OutputSizes=1
  Selector1 : Selector  IndexOptions=Index vector (dialog)  Indices=[6:13]  OutputSizes=1
  Selector2 : Selector  IndexOptions=Index vector (dialog)  Indices=[14:33]  OutputSizes=1
  Selector4 : Selector  IndexOptions=Index vector (dialog)  Indices=[34:41]  OutputSizes=1
  Sum : Sum  Inputs=|++
  p2m : Gain  Gain=1e6
  Out1 : Outport
  wires:
  Counter/1 -> Mux/5
  DOI_Main/1 -> Mux/1
  H2_Main/1 -> Mux/4
  SOI_Main/1 -> Mux/3
  In1/1 -> Selector4/1, Selector2/1, Selector1/1, Selector/1
  p2m/1 -> Mux/2
  Demux/1 -> Display2/1, DOI_Main/1
  Demux/2 -> Display1/1, p2m/1
  Demux/4 -> Display3/1, H2_Main/1
  Demux/5 -> Display4/1, Counter/1
  Demux/3 -> Display/1, Sum/1
  Sum/1 -> SOI_Main/1
  Constant/1 -> Sum/2
  Selector/1 -> Demux/1
  Gain/1 -> Add/1
  Constant1/1 -> Add/2
  Selector1/1 -> Gain/1
  Mux/1 -> Mux1/1
  Mux1/1 -> Out1/1
  Add/1 -> Saturation/1
  Saturation/1 -> Mux1/2
  Saturation1/1 -> Mux1/3
  Mux2/1 -> Add1/1
  Constant2/1 -> Add1/2
  Add1/1 -> Saturation1/1
  Selector2/1 -> Demux1/1
  Demux1/1 -> Gain2/1
  Demux1/2 -> Gain3/1
  Demux1/3 -> Gain4/1
  Demux1/4 -> Gain5/1
  Demux1/5 -> Gain6/1
  Demux1/6 -> Gain7/1
  Demux1/7 -> Gain8/1
  Demux1/8 -> Gain9/1
  Demux1/9 -> Gain10/1
  Demux1/10 -> Gain11/1
  Demux1/11 -> Gain12/1
  Demux1/12 -> Gain13/1
  Demux1/13 -> Gain14/1
  Demux1/14 -> Gain15/1
  Demux1/15 -> Gain16/1
  Demux1/16 -> Gain17/1
  Demux1/17 -> Gain18/1
  Demux1/18 -> Gain19/1
  Demux1/19 -> Gain20/1
  Demux1/20 -> Gain21/1
  Gain2/1 -> Mux2/1
  Gain3/1 -> Mux2/2
  Gain4/1 -> Mux2/3
  Gain5/1 -> Mux2/4
  Gain6/1 -> Mux2/5
  Gain7/1 -> Mux2/6
  Gain8/1 -> Mux2/7
  Gain9/1 -> Mux2/8
  Gain10/1 -> Mux2/9
  Gain11/1 -> Mux2/10
  Gain12/1 -> Mux2/11
  Gain13/1 -> Mux2/12
  Gain14/1 -> Mux2/13
  Gain16/1 -> Mux2/15
  Gain15/1 -> Mux2/14
  Gain17/1 -> Mux2/16
  Gain18/1 -> Mux2/17
  Gain19/1 -> Mux2/18
  Gain20/1 -> Mux2/19
  Gain21/1 -> Mux2/20
  Selector4/1 -> Demux2/1
  Demux2/1 -> Gain1/1
  Demux2/2 -> Gain22/1
  Demux2/3 -> Gain23/1
  Demux2/4 -> Gain24/1
  Gain1/1 -> Mux3/1
  Gain22/1 -> Mux3/2
  Gain23/1 -> Mux3/3
  Gain24/1 -> Mux3/4
  Saturation2/1 -> Mux1/4
  Mux3/1 -> Add2/1
  Constant3/1 -> Add2/2
  Add2/1 -> Saturation2/1
  Demux2/5 -> Gain25/1
  Demux2/6 -> Gain26/1
  Demux2/7 -> Gain27/1
  Demux2/8 -> Gain28/1
  Gain25/1 -> Mux3/5
  Gain26/1 -> Mux3/6
  Gain27/1 -> Mux3/7
  Gain28/1 -> Mux3/8

== system pi_IL_H2DF_2024a/main_C2C/main_C2C_n3/IL_Controller/Denorm_plant_IMEP_ref ==
  In : Inport
  Constant : Constant  Value=C2C_NMPC.Normalization.outputs.mean(1)
  Gain : Gain  Gain=C2C_NMPC.Normalization.outputs.std(1)
  Sum6 : Sum  Inputs=|++
  RefIn : Outport
  wires:
  In/1 -> Gain/1  "IMEP"
  Sum6/1 -> RefIn/1
  Gain/1 -> Sum6/1
  Constant/1 -> Sum6/2

== system pi_IL_H2DF_2024a/main_C2C/main_C2C_n3/IL_Controller/Denorm_plant_IMEP_ref1 ==
  In : Inport
  Constant : Constant  Value=C2C_NMPC.Normalization.outputs.mean(1)
  Gain : Gain  Gain=C2C_NMPC.Normalization.outputs.std(1)
  Sum6 : Sum  Inputs=|++
  RefIn : Outport
  wires:
  Constant/1 -> Sum6/2
  Gain/1 -> Sum6/1
  Sum6/1 -> RefIn/1
  In/1 -> Gain/1  "IMEP"

== system pi_IL_H2DF_2024a/main_C2C/main_C2C_n3/IL_Controller/IL_Controller_fb_FF_1 ==
  Ref : Inport
  feedback_load : Inport  Port=2
  Data Type Conversion : DataTypeConversion  OutDataTypeStr=double  SaturateOnIntegerOverflow=off  RndMeth=Floor
  Denorm_NN_Controls : Subsystem
  Mux : Mux  Inputs=2
  Norm_NN_IMEP_ref : Subsystem
  Norm_NN_IMEP_ref1 : Subsystem
  Predict : deeplib/Predict  Network=Network from MAT-file  NetworkFunction=squeezenet  NetworkFilePath=h2df_model_2024_0012_0008_0298.mat  MiniBatchSize=512  InputDataFormats={'',''}  Predictions=on  Activations={}  ForceInterpretedSim=off  EnableDLNetwork=on  LastKnownNetworkFilePath=''  LastKnownNetworkTimeStamp=''
  Control_norm_NN_params : Outport
  wires:
  Predict/1 -> Data Type Conversion/1
  Ref/1 -> Norm_NN_IMEP_ref/1(In)
  Data Type Conversion/1 -> Denorm_NN_Controls/1(controls_nn)  "Control_norm_NN_params"
  Mux/1 -> Predict/1
  Norm_NN_IMEP_ref/1(Out) -> Mux/1
  Norm_NN_IMEP_ref1/1(Out) -> Mux/2
  Denorm_NN_Controls/1(denorm_nn_u) -> Control_norm_NN_params/1
  feedback_load/1 -> Norm_NN_IMEP_ref1/1(In)

== system pi_IL_H2DF_2024a/main_C2C/main_C2C_n3/IL_Controller/Norm_Plant_Controls ==
  denorm_nn_u : Inport
  Constant10 : Constant  Value=C2C_NMPC.Normalization.controls.mean(2)
  Constant11 : Constant  Value=C2C_NMPC.Normalization.controls.mean(3)
  Constant12 : Constant  Value=C2C_NMPC.Normalization.controls.mean(4)
  Constant9 : Constant  Value=C2C_NMPC.Normalization.controls.mean(1)
  Demux : Demux
  Gain4 : Gain  Gain=1/C2C_NMPC.Normalization.controls.std(1)
  Gain5 : Gain  Gain=1/C2C_NMPC.Normalization.controls.std(2)
  Gain6 : Gain  Gain=1/C2C_NMPC.Normalization.controls.std(3)
  Gain7 : Gain  Gain=1/C2C_NMPC.Normalization.controls.std(4)
  Mux1 : Mux
  Sum{4,6..8} (4 alike) : Sum  Inputs=|+-
  controls : Outport
  wires:
  Mux1/1 -> controls/1
  denorm_nn_u/1 -> Demux/1
  Sum8/1 -> Gain7/1
  Demux/3 -> Sum7/1  "SOI_main"
  Constant12/1 -> Sum8/2
  Sum7/1 -> Gain6/1
  Constant11/1 -> Sum7/2
  Gain5/1 -> Mux1/2
  Gain4/1 -> Mux1/1
  Gain7/1 -> Mux1/4
  Demux/1 -> Sum4/1  "DOI_main"
  Constant9/1 -> Sum4/2
  Demux/2 -> Sum6/1  "SOI_pre"
  Sum4/1 -> Gain4/1
  Gain6/1 -> Mux1/3
  Constant10/1 -> Sum6/2
  Demux/4 -> Sum8/1  "DOI_H2"
  Sum6/1 -> Gain5/1

== system pi_IL_H2DF_2024a/main_C2C/main_C2C_n3/IL_Controller/SafetySaturation ==
  controls_nn_in : Inport
  Demux : Demux
  Mux : Mux
  Saturation : Saturate  UpperLimit=C2C_NMPC.Bounds.controls(1,2)  LowerLimit=C2C_NMPC.Bounds.controls(1,1)
  Saturation1 : Saturate  UpperLimit=C2C_NMPC.Bounds.controls(2,2)  LowerLimit=C2C_NMPC.Bounds.controls(2,1)
  Saturation2 : Saturate  UpperLimit=C2C_NMPC.Bounds.controls(3,2)  LowerLimit=C2C_NMPC.Bounds.controls(3,1)
  Saturation3 : Saturate  UpperLimit=C2C_NMPC.Bounds.controls(4,2)  LowerLimit=C2C_NMPC.Bounds.controls(4,1)
  controls_nn_out : Outport
  wires:
  controls_nn_in/1 -> Demux/1
  Demux/1 -> Saturation/1
  Demux/2 -> Saturation1/1
  Demux/3 -> Saturation2/1
  Demux/4 -> Saturation3/1
  Mux/1 -> controls_nn_out/1
  Saturation/1 -> Mux/1
  Saturation1/1 -> Mux/2
  Saturation2/1 -> Mux/3
  Saturation3/1 -> Mux/4

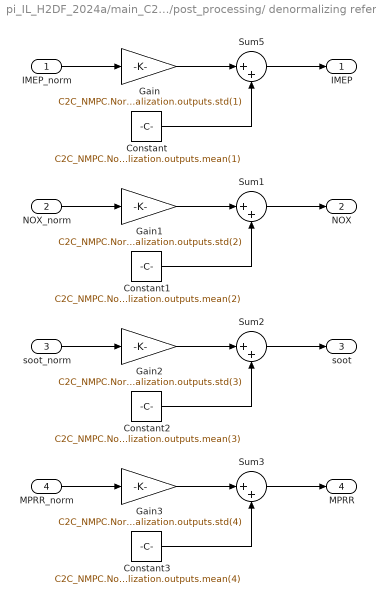
== system pi_IL_H2DF_2024a/main_C2C/main_C2C_n3/post_processing/ denormalizing reference ==
  IMEP_norm : Inport
  NOX_norm : Inport  Port=2
  soot_norm : Inport  Port=3
  MPRR_norm : Inport  Port=4
  Constant : Constant  Value=C2C_NMPC.Normalization.outputs.mean(1)
  Constant1 : Constant  Value=C2C_NMPC.Normalization.outputs.mean(2)
  Constant2 : Constant  Value=C2C_NMPC.Normalization.outputs.mean(3)
  Constant3 : Constant  Value=C2C_NMPC.Normalization.outputs.mean(4)
  Gain : Gain  Gain=C2C_NMPC.Normalization.outputs.std(1)
  Gain1 : Gain  Gain=C2C_NMPC.Normalization.outputs.std(2)
  Gain2 : Gain  Gain=C2C_NMPC.Normalization.outputs.std(3)
  Gain3 : Gain  Gain=C2C_NMPC.Normalization.outputs.std(4)
  Sum{1..3,5} (4 alike) : Sum  Inputs=|++
  IMEP : Outport
  NOX : Outport  Port=2
  soot : Outport  Port=3
  MPRR : Outport  Port=4
  wires:
  Gain/1 -> Sum5/1
  IMEP_norm/1 -> Gain/1
  Constant/1 -> Sum5/2
  Sum5/1 -> IMEP/1
  Gain1/1 -> Sum1/1
  Constant1/1 -> Sum1/2
  NOX_norm/1 -> Gain1/1
  Sum1/1 -> NOX/1
  Gain2/1 -> Sum2/1
  Constant2/1 -> Sum2/2
  soot_norm/1 -> Gain2/1
  Sum2/1 -> soot/1
  Gain3/1 -> Sum3/1
  Constant3/1 -> Sum3/2
  MPRR_norm/1 -> Gain3/1
  Sum3/1 -> MPRR/1

== system pi_IL_H2DF_2024a/main_C2C/main_C2C_n3/post_processing/Subsystem1 ==
  controller_ status : Inport
  Last_Output_MC : Inport  Port=2
  " denormalizing reference" : Subsystem
  Demux : Demux
  Mux : Mux
  Mux1 : Mux  Inputs=2
  Mux2 : Mux
  Selector1 : Selector  IndexOptions=Index vector (dialog)  Indices=[(4 + C2C_NMPC.Dims.n_controls * C2C_NMPC.Opts.N + 1 * (C2C_NMPC.Dims.n_states) + C2C_NMPC.Dims.n_LSTM_states + C2C_NMPC.Dims.n_controls +1):( 4 + C2C_NMPC.Dims.n_controls * C2C_NMPC.Opts.N + 2* C2C_NMPC.Dims.n_states)]  OutputSizes=1
  Selector2 : Selector  IndexOptions=Index vector (dialog)  Indices=[(4 + C2C_NMPC.Dims.n_controls * C2C_NMPC.Opts.N + 2 * (C2C_NMPC.Dims.n_states) + C2C_NMPC.Dims.n_LSTM_states + C2C_NMPC.Dims.n_controls +1):( 4 + C2C_NMPC.Dims.n_controls * C2C_NMPC.Opts.N + 3* C2C_NMPC.Dims.n_states)]  OutputSizes=1
  Selector3 : Selector  IndexOptions=Index vector (dialog)  Indices=[(4 + C2C_NMPC.Dims.n_controls * C2C_NMPC.Opts.N + 1* (C2C_NMPC.Dims.n_LSTM_states + C2C_NMPC.Dims.n_controls) +1) : (4 + C2C_NMPC.Dims.n_controls * C2C_NMPC.Opts.N + 1* C2C_NMPC.Dims.n_states)]  OutputSizes=1
  Selector4 : Selector  IndexOptions=Index vector (dialog)  Indices=[(4 + C2C_NMPC.Dims.n_controls * C2C_NMPC.Opts.N + 3 * (C2C_NMPC.Dims.n_states) + C2C_NMPC.Dims.n_LSTM_states + C2C_NMPC.Dims.n_controls +1):( 4 + C2C_NMPC.Dims.n_controls * C2C_NMPC.Opts.N + 4* C2C_NMPC.Dims.n_states)]  OutputSizes=1
  Subsystem : Subsystem
  Out1 : Outport
  wires:
  Last_Output_MC/1 -> Demux/1
  controller_ status/1 -> Selector4/1, Selector2/1, Selector1/1, Selector3/1
  Mux1/1 -> Out1/1
  Mux/1 -> Mux1/2
  Demux/1 -> " denormalizing reference"/1(IMEP_norm)
  Demux/2 -> " denormalizing reference"/2(NOX_norm)
  Demux/3 -> " denormalizing reference"/3(soot_norm)
  Demux/4 -> " denormalizing reference"/4(MPRR_norm)
  " denormalizing reference"/2(NOX) -> Mux2/2
  " denormalizing reference"/1(IMEP) -> Mux2/1
  " denormalizing reference"/3(soot) -> Mux2/3
  " denormalizing reference"/4(MPRR) -> Mux2/4
  Mux2/1 -> Mux1/1
  Subsystem/1(Node_0) -> Mux/1
  Selector3/1 -> Subsystem/1(In1)
  Selector1/1 -> Subsystem/2(In2)
  Subsystem/2(Node_1) -> Mux/2
  Subsystem/3(Node_2) -> Mux/3
  Subsystem/4(Node_3) -> Mux/4
  Selector4/1 -> Subsystem/4(In4)
  Selector2/1 -> Subsystem/3(In3)

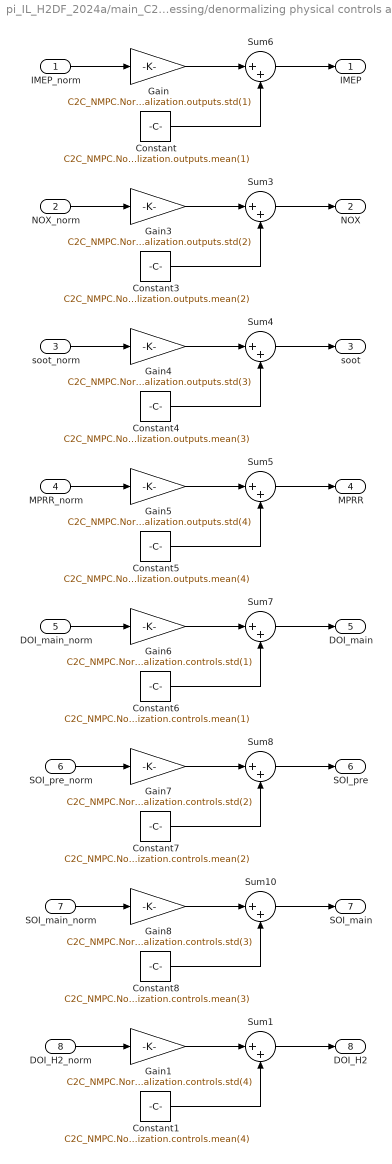
== system pi_IL_H2DF_2024a/main_C2C/main_C2C_n3/post_processing/denormalizing physical controls and outputs ==
  IMEP_norm : Inport
  NOX_norm : Inport  Port=2
  soot_norm : Inport  Port=3
  MPRR_norm : Inport  Port=4
  DOI_main_norm : Inport  Port=5
  SOI_pre_norm : Inport  Port=6
  SOI_main_norm : Inport  Port=7
  DOI_H2_norm : Inport  Port=8
  Constant : Constant  Value=C2C_NMPC.Normalization.outputs.mean(1)
  Constant1 : Constant  Value=C2C_NMPC.Normalization.controls.mean(4)
  Constant3 : Constant  Value=C2C_NMPC.Normalization.outputs.mean(2)
  Constant4 : Constant  Value=C2C_NMPC.Normalization.outputs.mean(3)
  Constant5 : Constant  Value=C2C_NMPC.Normalization.outputs.mean(4)
  Constant6 : Constant  Value=C2C_NMPC.Normalization.controls.mean(1)
  Constant7 : Constant  Value=C2C_NMPC.Normalization.controls.mean(2)
  Constant8 : Constant  Value=C2C_NMPC.Normalization.controls.mean(3)
  Gain : Gain  Gain=C2C_NMPC.Normalization.outputs.std(1)
  Gain1 : Gain  Gain=C2C_NMPC.Normalization.controls.std(4)
  Gain3 : Gain  Gain=C2C_NMPC.Normalization.outputs.std(2)
  Gain4 : Gain  Gain=C2C_NMPC.Normalization.outputs.std(3)
  Gain5 : Gain  Gain=C2C_NMPC.Normalization.outputs.std(4)
  Gain6 : Gain  Gain=C2C_NMPC.Normalization.controls.std(1)
  Gain7 : Gain  Gain=C2C_NMPC.Normalization.controls.std(2)
  Gain8 : Gain  Gain=C2C_NMPC.Normalization.controls.std(3)
  Sum{1,3..8,10} (8 alike) : Sum  Inputs=|++
  IMEP : Outport
  NOX : Outport  Port=2
  soot : Outport  Port=3
  MPRR : Outport  Port=4
  DOI_main : Outport  Port=5
  SOI_pre : Outport  Port=6
  SOI_main : Outport  Port=7
  DOI_H2 : Outport  Port=8
  wires:
  Gain4/1 -> Sum4/1
  Constant3/1 -> Sum3/2
  Constant4/1 -> Sum4/2
  Gain3/1 -> Sum3/1
  Constant5/1 -> Sum5/2
  Gain5/1 -> Sum5/1
  Constant/1 -> Sum6/2
  Sum3/1 -> NOX/1
  NOX_norm/1 -> Gain3/1
  Sum5/1 -> MPRR/1
  Gain/1 -> Sum6/1
  IMEP_norm/1 -> Gain/1
  Sum6/1 -> IMEP/1
  MPRR_norm/1 -> Gain5/1
  Sum4/1 -> soot/1
  soot_norm/1 -> Gain4/1
  Constant7/1 -> Sum8/2
  Gain8/1 -> Sum10/1
  Constant6/1 -> Sum7/2
  Gain7/1 -> Sum8/1
  Sum10/1 -> SOI_main/1
  DOI_main_norm/1 -> Gain6/1
  Sum7/1 -> DOI_main/1
  Gain6/1 -> Sum7/1
  Sum8/1 -> SOI_pre/1
  Constant8/1 -> Sum10/2
  SOI_main_norm/1 -> Gain8/1
  SOI_pre_norm/1 -> Gain7/1
  Sum1/1 -> DOI_H2/1
  Constant1/1 -> Sum1/2
  Gain1/1 -> Sum1/1
  DOI_H2_norm/1 -> Gain1/1

== system pi_IL_H2DF_2024a/main_C2C/main_C2C_n3/pre_processing1/normalize_last_outputs_MC ==
  data_in : Inport
  Constant : Constant  Value=C2C_NMPC.Normalization.outputs.mean(1)
  Constant1 : Constant  Value=C2C_NMPC.Normalization.outputs.mean(2)
  Constant2 : Constant  Value=C2C_NMPC.Normalization.outputs.mean(3)
  Constant3 : Constant  Value=C2C_NMPC.Normalization.outputs.mean(4)
  Demux : Demux
  Gain : Gain  Gain=1/C2C_NMPC.Normalization.outputs.std(1)
  Gain1 : Gain  Gain=1/C2C_NMPC.Normalization.outputs.std(2)
  Gain2 : Gain  Gain=1/C2C_NMPC.Normalization.outputs.std(3)
  Gain3 : Gain  Gain=1/C2C_NMPC.Normalization.outputs.std(4)
  Mux : Mux
  Selector1 : Selector  IndexOptions=Index vector (dialog)  Indices=[1:4]  OutputSizes=1
  Sum{1..3,5} (4 alike) : Sum  Inputs=|+-
  last_outputs_MC : Outport  VectorParamsAs1DForOutWhenUnconnected=off
  wires:
  Demux/2 -> Sum1/1
  Constant2/1 -> Sum2/2
  Sum2/1 -> Gain2/1
  Sum1/1 -> Gain1/1
  Gain3/1 -> Mux/4
  Gain1/1 -> Mux/2
  Constant1/1 -> Sum1/2
  Demux/3 -> Sum2/1
  Gain2/1 -> Mux/3
  Mux/1 -> last_outputs_MC/1
  Constant3/1 -> Sum3/2
  Sum3/1 -> Gain3/1
  Gain/1 -> Mux/1
  Sum5/1 -> Gain/1
  Constant/1 -> Sum5/2
  Demux/1 -> Sum5/1
  data_in/1 -> Selector1/1
  Demux/4 -> Sum3/1
  Selector1/1 -> Demux/1
